simulink model "problem4"  (R2020b)
settings: Solver=VariableStepAuto  StartTime=0.0  StopTime=10.0  RelTol=1e-3
settings Model: Creator=Shree  LastModifiedBy=Shree

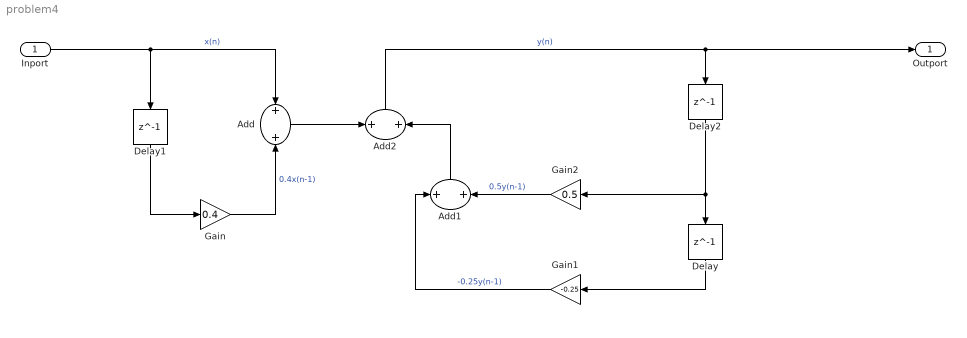
== system problem4 ==
  Inport : Inport
  Add : Sum
  Add1 : Sum
  Add2 : Sum
  Delay : Delay  DelayLength=1
  Delay1 : Delay  DelayLength=1
  Delay2 : Delay  DelayLength=1
  Gain : Gain  Gain=0.4
  Gain1 : Gain  Gain=-0.25
  Gain2 : Gain  Gain=0.5
  Outport : Outport
  wires:
  Inport/1 -> Delay1/1, Add/1  "x(n)"
  Delay1/1 -> Gain/1
  Gain/1 -> Add/2  "0.4x(n-1)"
  Add/1 -> Add2/1
  Add1/1 -> Add2/2
  Gain2/1 -> Add1/2  "0.5y(n-1)"
  Delay2/1 -> Gain2/1, Delay/1
  Add2/1 -> Outport/1, Delay2/1  "y(n)"
  Gain1/1 -> Add1/1  "-0.25y(n-1)"
  Delay/1 -> Gain1/1
